simulink model "D1"  (R2014b)
settings: Solver=ode45  StartTime=0.0  StopTime=1  RelTol=1e-3
undefined symbols (not defined in the file or in its folder): sigbuilder_block
settings Model: Creator=Emmanuel  LastModifiedBy=Emmanuel

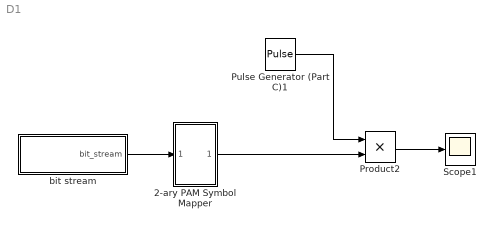
== system D1 ==
  2-ary PAM Symbol Mapper : Subsystem
  Product2 : Product
  Pulse Generator (Part C)1 : DiscretePulseGenerator  Period=50  PulseWidth=25  SampleTime=1/1000
  Scope1 : Scope
  bit stream : Subsystem  Tag=STV Subsys  LoadFcn=sigbuilder_block('load');  StartFcn=sigbuilder_block('start');  StopFcn=sigbuilder_block('stop');  ClipboardFcn=sigbuilder_block('clipboard');  mask(Sigbuilder block){}
      mask help: Simulink:masks:SigbuilderBlock_MD
      mask init:
      | if ~strcmp(get_param(bdroot(gcbh),'SimulationStatus'),'stopped') tuvar = sigbuilder_block('maskInit'); end
      settings: CopyFcn=sigbuilder_block('copy');  DeleteFcn=sigbuilder_block('delete');  ModelCloseFcn=sigbuilder_block('modelClose');  PreSaveFcn=sigbuilder_block('preSave');  PauseFcn=sigbuilder_block('pause');  ContinueFcn=sigbuilder_block('continue');  NameChangeFcn=sigbuilder_block('namechange');  OpenFcn=sigbuilder_block('open',[0 0 1440 754 ]);  CloseFcn=sigbuilder_block('close');
      mask Display: plot(0, 0, 100, 100,[2, 2, 32, 32, 2], [68, 8, 8, 68, 68],[32, 2], [38, 38], [32, 19, 2],[53, 60, 44], [32, 17, 17, 2],[16, 16, 31, 31]);txt = getActiveGroup(gcbh);text(2, 100, txt,'verticalAlignment', 'top');
  wires:
  Pulse Generator (Part C)1/1 -> Product2/1
  2-ary PAM Symbol Mapper/1(Out1) -> Product2/2
  Product2/1 -> Scope1/1
  bit stream/1(bit_stream) -> 2-ary PAM Symbol Mapper/1(In1)

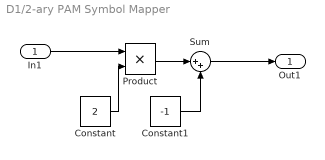
== system D1/2-ary PAM Symbol Mapper ==
  In1 : Inport
  Constant : Constant  Value=2  SampleTime=1/1000
  Constant1 : Constant  Value=-1  SampleTime=1/1000
  Product : Product
  Sum : Sum  Inputs=|++
  Out1 : Outport
  wires:
  Sum/1 -> Out1/1
  Constant1/1 -> Sum/2
  Product/1 -> Sum/1
  Constant/1 -> Product/2
  In1/1 -> Product/1

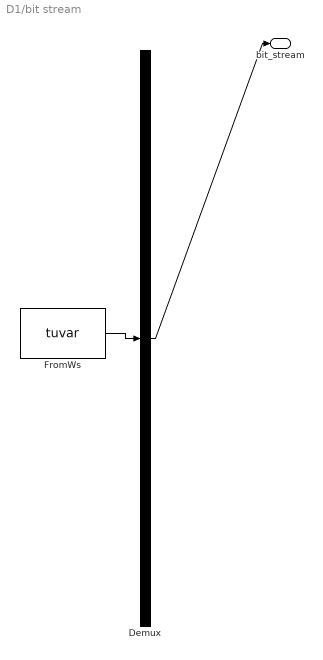
== system D1/bit stream ==
  Demux : Demux  Tag=STV Demux  Outputs=1
  FromWs : FromWorkspace  Tag=STV FromWs  VariableName=tuvar  SampleTime=1/1000
      SigBuilderData=|
      | common.afterFinalStr = 'Extrapolate'
      | common.sampleTime = '1/1000'
      | dataSet.timeRange = [0 1]
      | dataSet.name = ' '
      | sbobj.Groups.Name = ' '
      | sbobj.Groups.Signals.Name = 'bit_stream'
      | sbobj.Groups.Signals.XData = [0 0.1 0.1 0.3 0.3 0.5 0.6 0.6 0.9 0.9 1]
      | sbobj.Groups.Signals.YData = [1 1 0 0 1 1 1 0 0 1 1]
      | sbobj.Groups.TimeRange = [0 1]
  bit_stream : Outport  Tag=STV Outport
  wires:
  Demux/1 -> bit_stream/1
  FromWs/1 -> Demux/1
